simulink model "pmsm_control_sine"  (R2018b)
settings: Solver=VariableStepDiscrete  StartTime=0  StopTime=0.01  RelTol=1e-3
undefined symbols (not defined in the file or in its folder): DiscIntNeverNeededParam
libraries: powerlib x13, simulink x3, powerlib_meascontrol x2
settings Model: Creator=cemak  LastModifiedBy=canbe
settings DebuggingCC: LibraryContextMissingDiagnostic=none
settings SFSimCC: SimUseLocalCustomCode=off
settings RTWCC: RTWUseLocalCustomCode=off

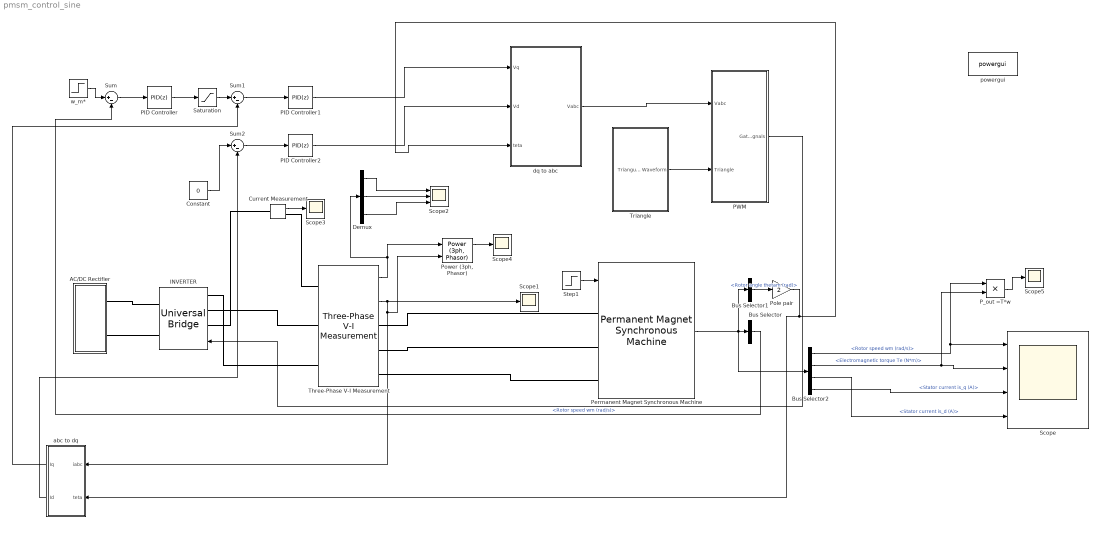
== system pmsm_control_sine ==
  AC/DC Rectifier : Subsystem
  Bus Selector : BusSelector  OutputSignals=Rotor speed wm (rad/s)
  Bus Selector1 : BusSelector  OutputSignals=Rotor angle thetam (rad)
  Bus Selector2 : BusSelector  OutputSignals=Rotor speed wm (rad/s),Electromagnetic torque Te (N*m),Stator current is_d (A),Stator current is_q (A)
  Constant : Constant  Value=0
  Current Measurement : powerlib/Measurements/Current Measurement  PhasorSimulation=off  OutputType=Complex  PSBequivalent=0
      settings: SourceProductName=Simscape Electrical
  Demux : Demux  Outputs=3
  INVERTER : powerlib/Power Electronics/Universal Bridge  Arms=3  SnubberResistance=1e5  SnubberCapacitance=inf  Device=IGBT / Diodes  Ron=1e-3  Lon=0  ForwardVoltages="[  5.8  1.55  ]"  ForwardVoltage=0  GTOparameters=[ 10e-6 , 20e-6 ]  IGBTparameters=[ 1e-6 , 2e-6 ]  Measurements=None  Measurements_2=None  converterType=Rectifier
      settings: SourceProductName=Simscape Electrical
  PID Controller : simulink/Continuous/PID Controller  Controller=PID  Form=Parallel  TimeDomain=Discrete-time  SampleTime=-1  IntegratorMethod=Forward Euler  FilterMethod=Forward Euler  ControllerParametersSource=internal  P=1000  I=10  D=0  UseFilter=on  N=100  TunerSelectOption=Transfer Function Based (PID Tuner App)  InitialConditionSource=internal  InitialConditionForIntegrator=0  InitialConditionForFilter=0  DifferentiatorICPrevScaledInput=0  ExternalReset=none  TrackingMode=off  Kt=1  LimitOutput=off  UpperSaturationLimit=inf  LowerSaturationLimit=-inf  LinearizeAsGain=on  AntiWindupMode=none  Kb=1  POutMin=[]  POutMax=[]  IOutMin=[]  IOutMax=[]  DOutMin=[]  DOutMax=[]  NOutMin=[]  NOutMax=[]  SumOutMin=[]  SumOutMax=[]  SaturationOutMin=[]  SaturationOutMax=[]  PParamMin=[]  PParamMax=[]  IParamMin=[]  IParamMax=[]  DParamMin=[]  DParamMax=[]  NParamMin=[]  NParamMax=[]  KbParamMin=[]  KbParamMax=[]  KtParamMin=[]  KtParamMax=[]  KbOutMin=[]  KbOutMax=[]  KtOutMin=[]  KtOutMax=[]  IntegratorOutMin=[]  IntegratorOutMax=[]  FilterOutMin=[]  FilterOutMax=[]  SumI1OutMin=[]  SumI1OutMax=[]  SumI2OutMin=[]  SumI2OutMax=[]  SumI3OutMin=[]  SumI3OutMax=[]  SumI4OutMin=[]  SumI4OutMax=[]  SumDOutMin=[]  SumDOutMax=[]  DifferentiatorOutMin=[]  DifferentiatorOutMax=[]  FilterDiffOutCoefMin=[]  FilterDiffOutCoefMax=[]  ReciprocalOutMin=[]  ReciprocalOutMax=[]  SumDenOutMin=[]  SumDenOutMax=[]  SumNumOutMin=[]  SumNumOutMax=[]  DivideOutMin=[]  DivideOutMax=[]  IntegratorContinuousStateAttributes=''  IntegratorStateMustResolveToSignalObject=off  IntegratorRTWStateStorageClass=Auto  FilterContinuousStateAttributes=''  FilterStateMustResolveToSignalObject=off  FilterRTWStateStorageClass=Auto  ParallelPVariant=InternalParameters  IdealPVariant=Disabled  IVariant=InternalParameters  DVariant=InternalParameters  IntegratorVariant=Discrete  SatVariant=Disabled  AWVariant=Passthrough  PCopyVariant=Disabled  TRVariant=Disabled  FdbkBlocksVariant=Forward  IdealPFdbkVariant=Disabled  SatFdbkVariant=Disabled  DerivativeFilterVariant=ForwardEulerFilter  NVariant=InternalParameters  NCopyVariant=Disabled  FilterICVariant=InternalICsFilter  IntegratorICVariant=InternalICs  ExternalResetVariant=Disabled  TRSumVariant=Passthrough  SumFdbkVariant=Disabled  SumVariant=Sum_PID
  PID Controller1 : simulink/Continuous/PID Controller  Controller=PID  Form=Parallel  TimeDomain=Discrete-time  SampleTime=-1  IntegratorMethod=Forward Euler  FilterMethod=Forward Euler  ControllerParametersSource=internal  P=2  I=1000  D=0  UseFilter=on  N=100  TunerSelectOption=Transfer Function Based (PID Tuner App)  InitialConditionSource=internal  InitialConditionForIntegrator=0  InitialConditionForFilter=0  DifferentiatorICPrevScaledInput=0  ExternalReset=none  TrackingMode=off  Kt=1  LimitOutput=off  UpperSaturationLimit=inf  LowerSaturationLimit=-inf  LinearizeAsGain=on  AntiWindupMode=none  Kb=1  POutMin=[]  POutMax=[]  IOutMin=[]  IOutMax=[]  DOutMin=[]  DOutMax=[]  NOutMin=[]  NOutMax=[]  SumOutMin=[]  SumOutMax=[]  SaturationOutMin=[]  SaturationOutMax=[]  PParamMin=[]  PParamMax=[]  IParamMin=[]  IParamMax=[]  DParamMin=[]  DParamMax=[]  NParamMin=[]  NParamMax=[]  KbParamMin=[]  KbParamMax=[]  KtParamMin=[]  KtParamMax=[]  KbOutMin=[]  KbOutMax=[]  KtOutMin=[]  KtOutMax=[]  IntegratorOutMin=[]  IntegratorOutMax=[]  FilterOutMin=[]  FilterOutMax=[]  SumI1OutMin=[]  SumI1OutMax=[]  SumI2OutMin=[]  SumI2OutMax=[]  SumI3OutMin=[]  SumI3OutMax=[]  SumI4OutMin=[]  SumI4OutMax=[]  SumDOutMin=[]  SumDOutMax=[]  DifferentiatorOutMin=[]  DifferentiatorOutMax=[]  FilterDiffOutCoefMin=[]  FilterDiffOutCoefMax=[]  ReciprocalOutMin=[]  ReciprocalOutMax=[]  SumDenOutMin=[]  SumDenOutMax=[]  SumNumOutMin=[]  SumNumOutMax=[]  DivideOutMin=[]  DivideOutMax=[]  IntegratorContinuousStateAttributes=''  IntegratorStateMustResolveToSignalObject=off  IntegratorRTWStateStorageClass=Auto  FilterContinuousStateAttributes=''  FilterStateMustResolveToSignalObject=off  FilterRTWStateStorageClass=Auto  ParallelPVariant=InternalParameters  IdealPVariant=Disabled  IVariant=InternalParameters  DVariant=InternalParameters  IntegratorVariant=Discrete  SatVariant=Disabled  AWVariant=Passthrough  PCopyVariant=Disabled  TRVariant=Disabled  FdbkBlocksVariant=Forward  IdealPFdbkVariant=Disabled  SatFdbkVariant=Disabled  DerivativeFilterVariant=ForwardEulerFilter  NVariant=InternalParameters  NCopyVariant=Disabled  FilterICVariant=InternalICsFilter  IntegratorICVariant=InternalICs  ExternalResetVariant=Disabled  TRSumVariant=Passthrough  SumFdbkVariant=Disabled  SumVariant=Sum_PID
  PID Controller2 : simulink/Continuous/PID Controller  Controller=PID  Form=Parallel  TimeDomain=Discrete-time  SampleTime=-1  IntegratorMethod=Forward Euler  FilterMethod=Forward Euler  ControllerParametersSource=internal  P=2  I=1000  D=0  UseFilter=on  N=100  TunerSelectOption=Transfer Function Based (PID Tuner App)  InitialConditionSource=internal  InitialConditionForIntegrator=0  InitialConditionForFilter=0  DifferentiatorICPrevScaledInput=0  ExternalReset=none  TrackingMode=off  Kt=1  LimitOutput=off  UpperSaturationLimit=inf  LowerSaturationLimit=-inf  LinearizeAsGain=on  AntiWindupMode=none  Kb=1  POutMin=[]  POutMax=[]  IOutMin=[]  IOutMax=[]  DOutMin=[]  DOutMax=[]  NOutMin=[]  NOutMax=[]  SumOutMin=[]  SumOutMax=[]  SaturationOutMin=[]  SaturationOutMax=[]  PParamMin=[]  PParamMax=[]  IParamMin=[]  IParamMax=[]  DParamMin=[]  DParamMax=[]  NParamMin=[]  NParamMax=[]  KbParamMin=[]  KbParamMax=[]  KtParamMin=[]  KtParamMax=[]  KbOutMin=[]  KbOutMax=[]  KtOutMin=[]  KtOutMax=[]  IntegratorOutMin=[]  IntegratorOutMax=[]  FilterOutMin=[]  FilterOutMax=[]  SumI1OutMin=[]  SumI1OutMax=[]  SumI2OutMin=[]  SumI2OutMax=[]  SumI3OutMin=[]  SumI3OutMax=[]  SumI4OutMin=[]  SumI4OutMax=[]  SumDOutMin=[]  SumDOutMax=[]  DifferentiatorOutMin=[]  DifferentiatorOutMax=[]  FilterDiffOutCoefMin=[]  FilterDiffOutCoefMax=[]  ReciprocalOutMin=[]  ReciprocalOutMax=[]  SumDenOutMin=[]  SumDenOutMax=[]  SumNumOutMin=[]  SumNumOutMax=[]  DivideOutMin=[]  DivideOutMax=[]  IntegratorContinuousStateAttributes=''  IntegratorStateMustResolveToSignalObject=off  IntegratorRTWStateStorageClass=Auto  FilterContinuousStateAttributes=''  FilterStateMustResolveToSignalObject=off  FilterRTWStateStorageClass=Auto  ParallelPVariant=InternalParameters  IdealPVariant=Disabled  IVariant=InternalParameters  DVariant=InternalParameters  IntegratorVariant=Discrete  SatVariant=Disabled  AWVariant=Passthrough  PCopyVariant=Disabled  TRVariant=Disabled  FdbkBlocksVariant=Forward  IdealPFdbkVariant=Disabled  SatFdbkVariant=Disabled  DerivativeFilterVariant=ForwardEulerFilter  NVariant=InternalParameters  NCopyVariant=Disabled  FilterICVariant=InternalICsFilter  IntegratorICVariant=InternalICs  ExternalResetVariant=Disabled  TRSumVariant=Passthrough  SumFdbkVariant=Disabled  SumVariant=Sum_PID
  PWM : Subsystem
  P_out =T*w : Product
  Permanent Magnet Synchronous Machine : powerlib/Machines/Permanent Magnet Synchronous Machine  NbPhases=3  FluxDistribution=Sinusoidal  RotorType=Salient-pole  MechanicalLoad=Torque Tm  PresetModel=No  ShowDetailedParameters=on  MeasurementBus=off  Resistance=16e-3  Inductance=8.5e-3  dqInductances=[350e-6 350e-6]  La=0.000395  MachineConstant=Flux linkage established by magnets (V.s)  Flux=0.5  VoltageCst=181.3799  TorqueCst=1.5  Flat=120  Mechanical=[10 0 2 0]  PolePairs=4  InitialConditions=[141.37 0 0,0]  InitialConditions5ph=[0 0 0 0 0 0]  TsPowergui=0  TsBlock=-1  RefAngle=90 degrees behind phase A axis (modified Park)
  "Pole pair " : Gain  Gain=2
  "Power (3ph, Phasor)" : powerlib_meascontrol/Measurements/Power (3ph, Phasor)
      settings: SourceProductName=Simscape Electrical  SourceProductBaseCode=PS
  Saturation : Saturate  UpperLimit=229  LowerLimit=-229
  Scope : Scope  NumInputPorts=4
  Scope{1,3..5} (4 alike) : Scope
  Scope2 : Scope  NumInputPorts=3
  Step1 : Step  Time=2  After=0  SampleTime=0
  Sum : Sum  Inputs=|+-
  Sum1 : Sum  Inputs=|+-
  Sum2 : Sum  Inputs=|+-
  Three-Phase V-I Measurement : powerlib/Measurements/Three-Phase V-I Measurement  VoltageMeasurement=phase-to-phase  SetLabelV=off  LabelV=Vabc  Vpu=off  VpuLL=off  CurrentMeasurement=yes  SetLabelI=off  LabelI=Iabc  Ipu=off  Pbase=100e6  Vbase=500e3  OutputType=Complex  PhasorSimulation=off  PSBequivalent=0
      settings: SourceProductName=Simscape Electrical
  Triangle : Subsystem
  abc to dq : Subsystem
  dq to abc : Subsystem
  powergui : powerlib/powergui  Priority=1  SimulationMode=Discrete  SampleTime=1e-8  frequency=60  Iterations=50  frequencyindice=0  Pbase=100e6  ErrMax=1e-4  UnitsV=kV  UnitsW=MW  buscounter=0  FunctionMessages=off  echomessages=off  EnableUseOfTLC=off  CurrentSourceSwitches=off  DisableSnubberDevices=off  DisableRonSwitches=off  DisableVfSwitches=off  DisplayEquations=off  SolverType=Tustin/Backward Euler (TBE)  Interpol=off  ExternalGateDelay=off  methode=off  Ts=100  x0status=blocks  SPID=on  SwTol=0  HookPort=off  RestoreLinks=warning  ResistiveCurrentMeasurement=off  Frange=[0:2:500]  Ylog=off  Xlog=on  ShowGrid=off  save=off  variable=ZData  structure=0  ZoomFFT=off  StartTime=0.0  cycles=1  DisplayStyle=1  fundamental=60  FreqAxis=off  MaxFrequency=1000  frequencyindicesteady=1  RmsSteady=1  display=off
  "w_m* " : Step  Time=0.5  Before=266.6  After=-266.6  SampleTime=0
  wires:
  Sum/1 -> PID Controller/1
  "w_m* "/1 -> Sum/1
  PID Controller/1 -> Saturation/1
  Permanent Magnet Synchronous Machine/1 -> Bus Selector2/1, Bus Selector1/1, Bus Selector/1
  Bus Selector/1 -> Sum/2  "<Rotor speed wm (rad/s)>"
  Bus Selector1/1 -> "Pole pair "/1  "<Rotor angle thetam (rad)>"
  Bus Selector2/1 -> P_out =T*w/1, Scope/1  "<Rotor speed wm (rad/s)>"
  Bus Selector2/2 -> Scope/2, P_out =T*w/2  "<Electromagnetic torque Te (N*m)>"
  Step1/1 -> Permanent Magnet Synchronous Machine/1
  Saturation/1 -> Sum1/1
  Sum1/1 -> PID Controller1/1
  Constant/1 -> Sum2/1
  PID Controller1/1 -> dq to abc/1(Vq)
  "Pole pair "/1 -> abc to dq/2(teta), dq to abc/3(teta)
  dq to abc/1(Vabc) -> PWM/1("Vabc ")
  Three-Phase V-I Measurement/2 -> abc to dq/1(iabc), "Power (3ph, Phasor)"/2, Scope1/1
  abc to dq/1(Iq) -> Sum1/2
  abc to dq/2(Id) -> Sum2/2
  Three-Phase V-I Measurement/1 -> "Power (3ph, Phasor)"/1, Demux/1
  Demux/1 -> Scope2/1
  Demux/2 -> Scope2/2
  Demux/3 -> Scope2/3
  Bus Selector2/4 -> Scope/3  "<Stator current is_q (A)>"
  Bus Selector2/3 -> Scope/4  "<Stator current is_d (A)>"
  Sum2/1 -> PID Controller2/1
  PID Controller2/1 -> dq to abc/2(Vd)
  Current Measurement/1 -> Scope3/1
  "Power (3ph, Phasor)"/1 -> Scope4/1
  P_out =T*w/1 -> Scope5/1
  PWM/1(Gate Signals) -> INVERTER/1
  Triangle/1(Triangular Waveform) -> PWM/2("Triangle ")
  connections:
  INVERTER/LConn2 -- Three-Phase V-I Measurement/LConn2
  INVERTER/LConn3 -- Three-Phase V-I Measurement/LConn3
  Three-Phase V-I Measurement/RConn1 -- Permanent Magnet Synchronous Machine/LConn1
  Three-Phase V-I Measurement/RConn2 -- Permanent Magnet Synchronous Machine/LConn2
  Three-Phase V-I Measurement/RConn3 -- Permanent Magnet Synchronous Machine/LConn3
  AC/DC Rectifier/LConn1 -- INVERTER/RConn2
  INVERTER/LConn1 -- Current Measurement/LConn1
  Current Measurement/RConn1 -- Three-Phase V-I Measurement/LConn1
  AC/DC Rectifier/LConn2 -- INVERTER/RConn1

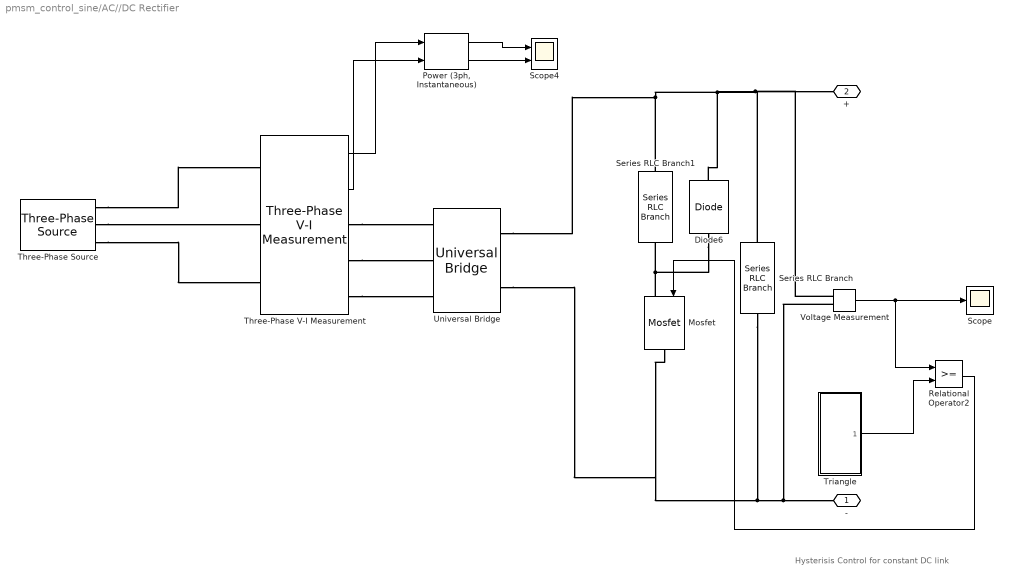
== system pmsm_control_sine/AC//DC Rectifier ==
  note: Hysterisis Control for constant DC link
  Diode6 : powerlib/Power Electronics/Diode  Ron=0.001  Lon=0  Vf=1  IC=0  UseSnubber=0  Rs=500  Cs=250e-9  Measurements=off
      settings: SourceProductName=Simscape Electrical
  Mosfet : powerlib/Power Electronics/Mosfet  Ron=0.1  Lon=0  Rd=0.025  Vfd=0  IC=0  Rs=1e5  Cs=inf  Measurements=off
      settings: SourceProductName=Simscape Electrical
  "Power (3ph, Instantaneous)" : powerlib_meascontrol/Measurements/Power (3ph, Instantaneous)
      settings: SourceProductName=Simscape Electrical
  Relational Operator2 : RelationalOperator  OutDataTypeStr=boolean  RndMeth=Simplest
  Scope : Scope
  Scope4 : Scope  NumInputPorts=2
  Series RLC Branch : powerlib/Elements/Series RLC Branch  LConnTagsString=__new0  RConnTagsString=__new0  BranchType=C  Resistance=1  Inductance=1e-3  SetiL0=off  InitialCurrent=0  Capacitance=990e-6  Setx0=off  InitialVoltage=0  Measurements=None
      settings: SourceProductName=Simscape Electrical
  Series RLC Branch1 : powerlib/Elements/Series RLC Branch  LConnTagsString=__new0  RConnTagsString=__new0  BranchType=R  Resistance=4.5  Inductance=1e-3  SetiL0=off  InitialCurrent=0  Capacitance=1e-6  Setx0=off  InitialVoltage=0  Measurements=None
      settings: SourceProductName=Simscape Electrical
  Three-Phase V-I Measurement : powerlib/Measurements/Three-Phase V-I Measurement  VoltageMeasurement=phase-to-phase  SetLabelV=off  LabelV=Vabc  Vpu=off  VpuLL=off  CurrentMeasurement=yes  SetLabelI=off  LabelI=Iabc  Ipu=off  Pbase=100e6  Vbase=500e3  OutputType=Complex  PhasorSimulation=off  PSBequivalent=0
      settings: SourceProductName=Simscape Electrical
  Three-Phase Source : powerlib/Electrical Sources/Three-Phase Source  InternalConnection=Y  VoltagePhases=off  Voltage=400  PhaseAngle=0  Voltage_phases=[25e3 25e3 25e3]/sqrt(3)  PhaseAngles_phases=[0 -120 +120]  Frequency=50  NonIdealSource=off  SpecifyImpedance=off  Resistance=0.8929  Inductance=16.58e-3  ShortCircuitLevel=100e6  BaseVoltage=25e3  XRratio=7  BusType=swing  Pref=10e3  Qref=0  Prefabc=[10e3, 10e3, 10e3]  Qrefabc=[0, 0, 0]  Qmin=-inf  Qmax=inf
      settings: SourceProductName=Simscape Electrical
  Triangle : Subsystem
  Universal Bridge : powerlib/Power Electronics/Universal Bridge  Arms=3  SnubberResistance=1e5  SnubberCapacitance=inf  Device=Diodes  Ron=1e-3  Lon=0  ForwardVoltages="[  0  0  ]"  ForwardVoltage=1.31  GTOparameters=[ 10e-6 , 20e-6 ]  IGBTparameters=[ 1e-6 , 2e-6 ]  Measurements=None  Measurements_2=None  converterType=Rectifier
      settings: SourceProductName=Simscape Electrical
  Voltage Measurement : powerlib/Measurements/Voltage Measurement  PhasorSimulation=off  OutputType=Complex  PSBequivalent=0
      settings: SourceProductName=Simscape Electrical
  - : PMIOPort  Side=Left
  + : PMIOPort  Port=2  Side=Left
  wires:
  Triangle/1(Triangular) -> Relational Operator2/2
  Voltage Measurement/1 -> Scope/1, Relational Operator2/1
  Three-Phase V-I Measurement/1 -> "Power (3ph, Instantaneous)"/1
  Three-Phase V-I Measurement/2 -> "Power (3ph, Instantaneous)"/2
  "Power (3ph, Instantaneous)"/1 -> Scope4/1
  Relational Operator2/1 -> Mosfet/1
  "Power (3ph, Instantaneous)"/2 -> Scope4/2
  connections:
  Series RLC Branch/LConn1 -- Voltage Measurement/LConn1 -- +/RConn1 -- Diode6/RConn1 -- Universal Bridge/RConn1 -- Series RLC Branch1/LConn1
  Mosfet/LConn1 -- Diode6/LConn1 -- Series RLC Branch1/RConn1
  Universal Bridge/RConn2 -- Mosfet/RConn1 -- Series RLC Branch/RConn1 -- Voltage Measurement/LConn2 -- -/RConn1
  Three-Phase V-I Measurement/RConn1 -- Universal Bridge/LConn1
  Three-Phase V-I Measurement/RConn2 -- Universal Bridge/LConn2
  Three-Phase V-I Measurement/RConn3 -- Universal Bridge/LConn3
  Three-Phase Source/RConn1 -- Three-Phase V-I Measurement/LConn1
  Three-Phase Source/RConn2 -- Three-Phase V-I Measurement/LConn2
  Three-Phase Source/RConn3 -- Three-Phase V-I Measurement/LConn3

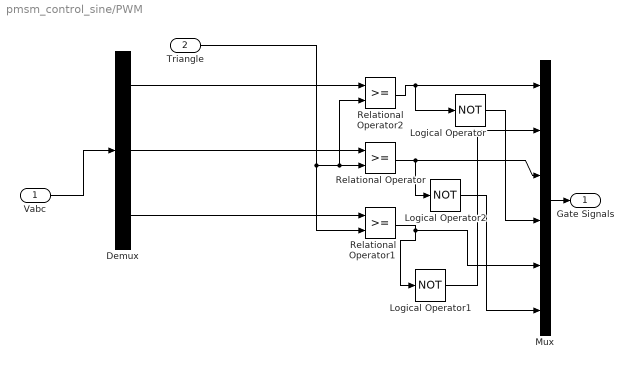
== system pmsm_control_sine/PWM ==
  "Vabc " : Inport
  "Triangle " : Inport  Port=2
  Demux : Demux  Outputs=3
  Logical Operator : Logic  Operator=NOT  AllPortsSameDT=off  OutDataTypeStr=boolean
  Logical Operator1 : Logic  Operator=NOT  AllPortsSameDT=off  OutDataTypeStr=boolean
  Logical Operator2 : Logic  Operator=NOT  AllPortsSameDT=off  OutDataTypeStr=boolean
  Mux : Mux  Inputs=6
  Relational Operator : RelationalOperator  OutDataTypeStr=boolean  RndMeth=Simplest
  Relational Operator1 : RelationalOperator  OutDataTypeStr=boolean  RndMeth=Simplest
  Relational Operator2 : RelationalOperator  OutDataTypeStr=boolean  RndMeth=Simplest
  Gate Signals : Outport
  wires:
  Relational Operator1/1 -> Logical Operator1/1, Mux/5
  Mux/1 -> Gate Signals/1
  Demux/2 -> Relational Operator/1
  Relational Operator2/1 -> Logical Operator/1, Mux/1
  Relational Operator/1 -> Logical Operator2/1, Mux/3
  Demux/3 -> Relational Operator1/1
  Demux/1 -> Relational Operator2/1
  "Vabc "/1 -> Demux/1
  "Triangle "/1 -> Relational Operator1/2, Relational Operator2/2, Relational Operator/2
  Logical Operator/1 -> Mux/4
  Logical Operator2/1 -> Mux/6
  Logical Operator1/1 -> Mux/2

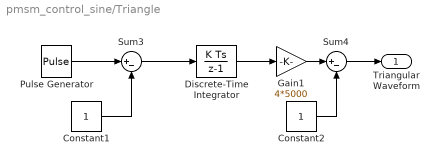
== system pmsm_control_sine/Triangle ==
  Constant1 : Constant
  Constant2 : Constant
  Discrete-Time Integrator : DiscreteIntegrator  SampleTime=-1  ICPrevOutput=DiscIntNeverNeededParam  ICPrevScaledInput=DiscIntNeverNeededParam
  Gain1 : Gain  Gain=4*5000
  Pulse Generator : DiscretePulseGenerator  PulseType=Time based  Amplitude=2  Period=1/5000  PulseWidth=50
  Sum3 : Sum  Inputs=|+-
  Sum4 : Sum  Inputs=|+-
  Triangular Waveform : Outport
  wires:
  Constant1/1 -> Sum3/2
  Gain1/1 -> Sum4/1
  Constant2/1 -> Sum4/2
  Sum4/1 -> Triangular Waveform/1
  Sum3/1 -> Discrete-Time Integrator/1
  Pulse Generator/1 -> Sum3/1
  Discrete-Time Integrator/1 -> Gain1/1

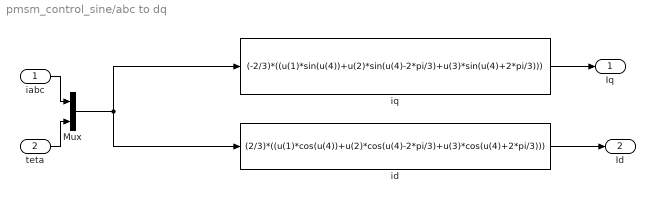
== system pmsm_control_sine/abc to dq ==
  iabc : Inport
  teta : Inport  Port=2
  Mux : Mux  Inputs=2
  id : Fcn  Expr=(2/3)*((u(1)*cos(u(4))+u(2)*cos(u(4)-2*pi/3)+u(3)*cos(u(4)+2*pi/3)))
  iq : Fcn  Expr=(-2/3)*((u(1)*sin(u(4))+u(2)*sin(u(4)-2*pi/3)+u(3)*sin(u(4)+2*pi/3)))
  Iq : Outport
  Id : Outport  Port=2
  wires:
  Mux/1 -> id/1, iq/1
  id/1 -> Id/1
  iabc/1 -> Mux/1
  teta/1 -> Mux/2
  iq/1 -> Iq/1

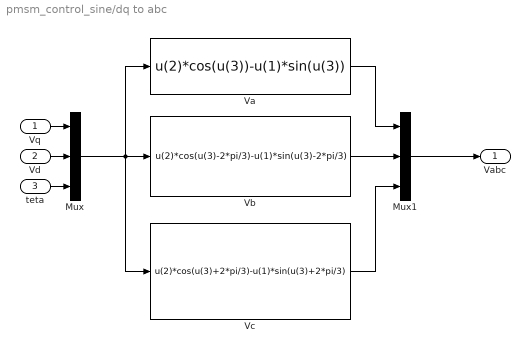
== system pmsm_control_sine/dq to abc ==
  Vq : Inport
  Vd : Inport  Port=2
  teta : Inport  Port=3
  Mux : Mux  Inputs=3
  Mux1 : Mux  Inputs=3
  Va : Fcn  Expr=u(2)*cos(u(3))-u(1)*sin(u(3))
  Vb : Fcn  Expr=u(2)*cos(u(3)-2*pi/3)-u(1)*sin(u(3)-2*pi/3)
  "Vc " : Fcn  Expr=u(2)*cos(u(3)+2*pi/3)-u(1)*sin(u(3)+2*pi/3)
  Vabc : Outport
  wires:
  Vq/1 -> Mux/1
  Va/1 -> Mux1/1
  Mux/1 -> Va/1, Vb/1, "Vc "/1
  Vd/1 -> Mux/2
  "Vc "/1 -> Mux1/3
  Vb/1 -> Mux1/2
  teta/1 -> Mux/3
  Mux1/1 -> Vabc/1

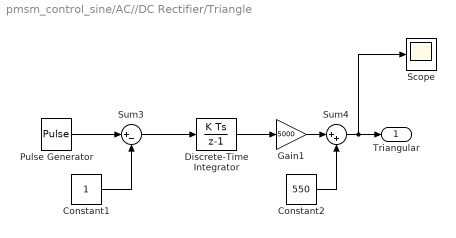
== system pmsm_control_sine/AC//DC Rectifier/Triangle ==
  Constant1 : Constant
  Constant2 : Constant  Value=550
  Discrete-Time Integrator : DiscreteIntegrator  SampleTime=-1  ICPrevOutput=DiscIntNeverNeededParam  ICPrevScaledInput=DiscIntNeverNeededParam
  Gain1 : Gain  Gain=5000
  Pulse Generator : DiscretePulseGenerator  PulseType=Time based  Amplitude=2  Period=1/5000  PulseWidth=50
  Scope : Scope
  Sum3 : Sum  Inputs=|+-
  Sum4 : Sum  Inputs=|++
  Triangular : Outport
  wires:
  Constant1/1 -> Sum3/2
  Gain1/1 -> Sum4/1
  Constant2/1 -> Sum4/2
  Sum4/1 -> Scope/1, Triangular/1
  Sum3/1 -> Discrete-Time Integrator/1
  Pulse Generator/1 -> Sum3/1
  Discrete-Time Integrator/1 -> Gain1/1
